simulink model "BodyMPC"  (R2023b)
settings: Solver=daessc  StartTime=0.0  StopTime=10  FixedStep=0.01  RelTol=1e-3
values from neighbouring files (symbols this model uses):
  Q = blkdiag(Q, q)    [SolveMPC.m]
undefined symbols (not defined in the file or in its folder): dw_des, LFstates, LRstates, p_cur, p_des, px, py, pz, RFstates, RRstates, v_cur, v_des, vx, vy, vz, w, w_des, X, Y, Z
libraries: sm_lib x57, nesl_utility x47
(part 1 of 3)
settings Model: Creator=a123  LastModifiedBy=a123

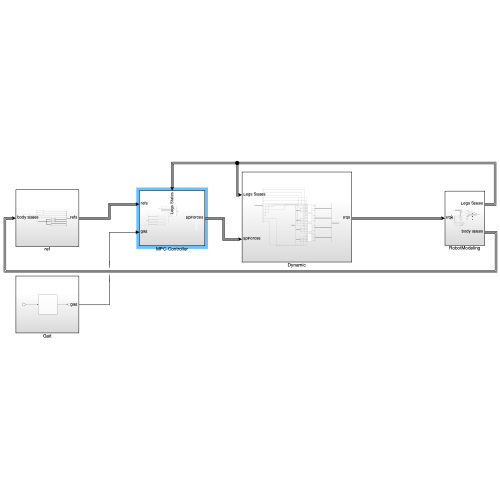
[thumbnail: Simulink's stored preview of the top-level diagram]
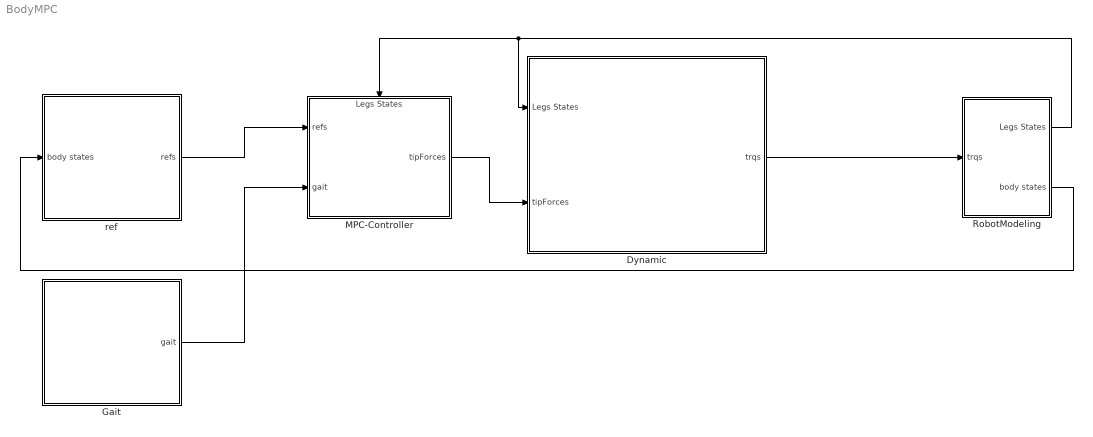
== system BodyMPC ==
  Dynamic : Subsystem
  Gait : Subsystem
  MPC-Controller : Subsystem
      settings: PortSchema="{\"entries\":[{\"content\":{\"sides\":[{\"content\":{\"connectorIds\":[\"In1\",\"In2\"]},\"type\":\"ConnectorPlacement.EquallySpacedRectSide\",\"uuid\":\"82207ac2-498d-428d-bb4d-b0457fff2070\"},{\"content\":{\"connectorIds\":[\"Out1\"],\"side\":\"RIGHT\"},\"type\":\"ConnectorPlacement.EquallySpacedRectSide\",\"uuid\":\"62017463-8491-4b37-95c8-f619666068a7\"},{\"content\":{\"connectorIds\":[\"In3\"],\"side\":\"TOP\"},\"type\":\"ConnectorPlacement.EquallySpacedRectSide\",\"uuid\":\"cf9993cf-df0f-41a3-a963-d91c0f700b7a\"}]},\"type\":\"ConnectorPlacement.EquallySpacedConnector\",\"uuid\":\"3cbcd1c8-4438-4464-bb77-c195fb75fbb3\"}],\"packageUris\":[\"http://schema.mathworks.com/mf0/Connector/R2020b\"],\"version\":\"1.0\"}"
  RobotModeling : Subsystem
  ref : Subsystem
  wires:
  RobotModeling/2(" body states") -> ref/1(body states)
  Dynamic/1(trqs) -> RobotModeling/1(trqs)
  RobotModeling/1(Legs States) -> MPC-Controller/3(Legs States), Dynamic/1(Legs States)
  ref/1(refs) -> MPC-Controller/1(refs)
  Gait/1(gait) -> MPC-Controller/2(gait)
  MPC-Controller/1(tipForces) -> Dynamic/2(tipForces)

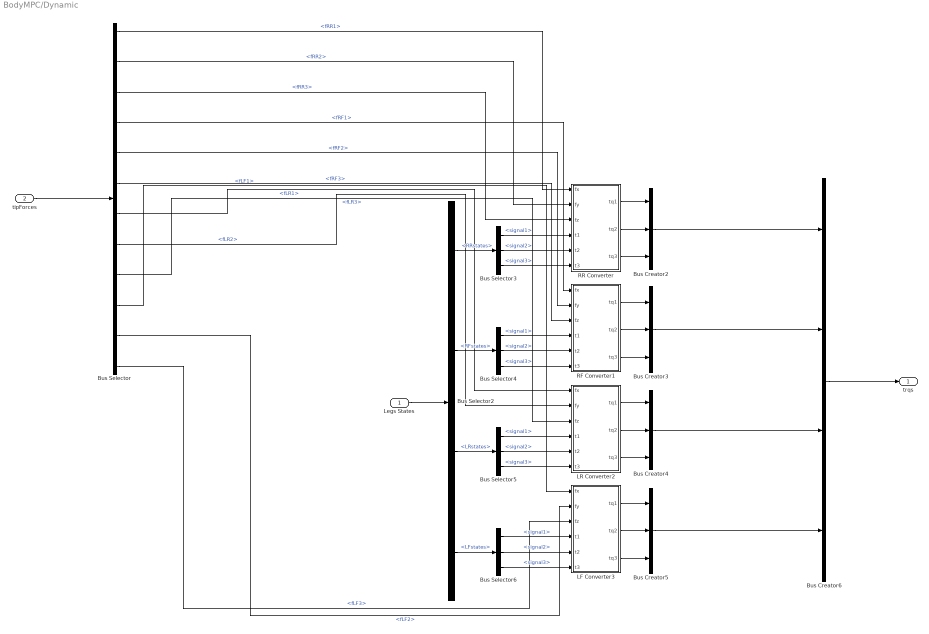
== system BodyMPC/Dynamic ==
  Legs States : Inport
  tipForces : Inport  Port=2
  Bus Creator{2..5} (4 alike) : BusCreator  Inputs=3
  Bus Creator6 : BusCreator  Inputs=4
  Bus Selector : BusSelector  OutputSignals=fRR1,fRR2,fRR3,fRF1,fRF2,fRF3,fLR1,fLR2,fLR3,fLF1,fLF2,fLF3
  Bus Selector2 : BusSelector  OutputSignals=RRstates,RFstates,LRstates,LFstates
  Bus Selector{3..6} (4 alike) : BusSelector  OutputSignals=signal1,signal2,signal3
  LF Converter3 : MATLAB Function  TreatAsAtomicUnit=on
  LR Converter2 : MATLAB Function  TreatAsAtomicUnit=on
  RF Converter1 : MATLAB Function  TreatAsAtomicUnit=on
  RR Converter : MATLAB Function  TreatAsAtomicUnit=on
  trqs : Outport
  wires:
  Bus Creator2/1 -> Bus Creator6/1
  Bus Creator3/1 -> Bus Creator6/2
  Bus Creator4/1 -> Bus Creator6/3
  Bus Creator5/1 -> Bus Creator6/4
  Bus Creator6/1 -> trqs/1
  Legs States/1 -> Bus Selector2/1
  Bus Selector2/1 -> Bus Selector3/1  "<RRstates>"
  Bus Selector3/1 -> RR Converter/4(t1)  "<signal1>"
  Bus Selector3/2 -> RR Converter/5(t2)  "<signal2>"
  Bus Selector3/3 -> RR Converter/6(t3)  "<signal3>"
  Bus Selector2/2 -> Bus Selector4/1  "<RFstates>"
  Bus Selector2/3 -> Bus Selector5/1  "<LRstates>"
  Bus Selector2/4 -> Bus Selector6/1  "<LFstates>"
  Bus Selector4/1 -> RF Converter1/4(t1)  "<signal1>"
  Bus Selector4/2 -> RF Converter1/5(t2)  "<signal2>"
  Bus Selector4/3 -> RF Converter1/6(t3)  "<signal3>"
  Bus Selector5/1 -> LR Converter2/4(t1)  "<signal1>"
  Bus Selector5/2 -> LR Converter2/5(t2)  "<signal2>"
  Bus Selector5/3 -> LR Converter2/6(t3)  "<signal3>"
  Bus Selector6/1 -> LF Converter3/4(t1)  "<signal1>"
  Bus Selector6/2 -> LF Converter3/5(t2)  "<signal2>"
  Bus Selector6/3 -> LF Converter3/6(t3)  "<signal3>"
  RR Converter/3(tq3) -> Bus Creator2/3
  RR Converter/2(tq2) -> Bus Creator2/2
  RR Converter/1(tq1) -> Bus Creator2/1
  RF Converter1/1(tq1) -> Bus Creator3/1
  RF Converter1/2(tq2) -> Bus Creator3/2
  RF Converter1/3(tq3) -> Bus Creator3/3
  LR Converter2/1(tq1) -> Bus Creator4/1
  LR Converter2/2(tq2) -> Bus Creator4/2
  LR Converter2/3(tq3) -> Bus Creator4/3
  LF Converter3/1(tq1) -> Bus Creator5/1
  LF Converter3/2(tq2) -> Bus Creator5/2
  LF Converter3/3(tq3) -> Bus Creator5/3
  tipForces/1 -> Bus Selector/1
  Bus Selector/1 -> RR Converter/1(fx)  "<fRR1>"
  Bus Selector/2 -> RR Converter/2(fy)  "<fRR2>"
  Bus Selector/3 -> RR Converter/3(fz)  "<fRR3>"
  Bus Selector/4 -> RF Converter1/1(fx)  "<fRF1>"
  Bus Selector/5 -> RF Converter1/2(fy)  "<fRF2>"
  Bus Selector/6 -> RF Converter1/3(fz)  "<fRF3>"
  Bus Selector/7 -> LR Converter2/1(fx)  "<fLR1>"
  Bus Selector/8 -> LR Converter2/2(fy)  "<fLR2>"
  Bus Selector/9 -> LR Converter2/3(fz)  "<fLR3>"
  Bus Selector/10 -> LF Converter3/1(fx)  "<fLF1>"
  Bus Selector/11 -> LF Converter3/2(fy)  "<fLF2>"
  Bus Selector/12 -> LF Converter3/3(fz)  "<fLF3>"

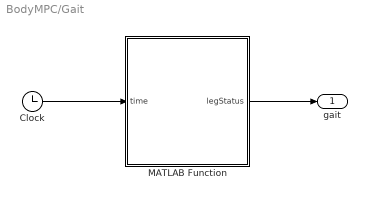
== system BodyMPC/Gait ==
  Clock : Clock
  MATLAB Function : MATLAB Function  TreatAsAtomicUnit=on
  gait : Outport
  wires:
  Clock/1 -> MATLAB Function/1(time)
  MATLAB Function/1(legStatus) -> gait/1

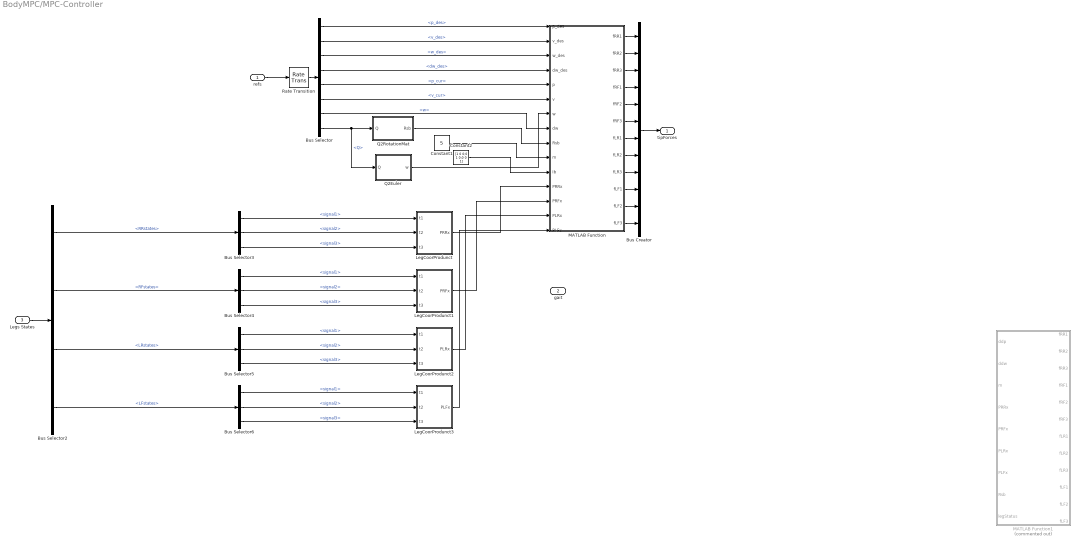
== system BodyMPC/MPC-Controller ==
  refs : Inport
  gait : Inport  Port=2
  Legs States : Inport  Port=3
  Bus Creator : BusCreator  Inputs=12
  Bus Selector : BusSelector  OutputSignals=p_des,v_des,w_des,dw_des,p_cur,v_cur,w,Q
  Bus Selector2 : BusSelector  OutputSignals=RRstates,RFstates,LRstates,LFstates
  Bus Selector{3..6} (4 alike) : BusSelector  OutputSignals=signal1,signal2,signal3
  Constant1 : Constant  Value=5
  Constant2 : Constant  Value=[1 0 0;0 1 0;0 0 1]
  LegCoorProdunct : MATLAB Function  TreatAsAtomicUnit=on
  LegCoorProdunct1 : MATLAB Function  TreatAsAtomicUnit=on
  LegCoorProdunct2 : MATLAB Function  TreatAsAtomicUnit=on
  LegCoorProdunct3 : MATLAB Function  TreatAsAtomicUnit=on
  MATLAB Function : MATLAB Function  TreatAsAtomicUnit=on
  MATLAB Function1 : MATLAB Function  Commented=on  TreatAsAtomicUnit=on
  Q2Euler : MATLAB Function  TreatAsAtomicUnit=on
  Q2RotationMat : MATLAB Function  TreatAsAtomicUnit=on
  Rate Transition : RateTransition  OutPortSampleTime=0.001
  tipForces : Outport
  wires:
  refs/1 -> Rate Transition/1
  Bus Selector/1 -> MATLAB Function/1(p_des)  "<p_des>"
  Bus Selector/2 -> MATLAB Function/2(v_des)  "<v_des>"
  Bus Selector/3 -> MATLAB Function/3(w_des)  "<w_des>"
  Bus Selector/4 -> MATLAB Function/4(dw_des)  "<dw_des>"
  Bus Selector/5 -> MATLAB Function/5(p)  "<p_cur>"
  Bus Selector/6 -> MATLAB Function/6(v)  "<v_cur>"
  Bus Selector/7 -> MATLAB Function/8(dw)  "<w>"
  Bus Selector/8 -> Q2Euler/1(Q), Q2RotationMat/1(Q)  "<Q>"
  Bus Selector5/2 -> LegCoorProdunct2/2(t2)  "<signal2>"
  Bus Selector5/3 -> LegCoorProdunct2/3(t3)  "<signal3>"
  Bus Selector6/3 -> LegCoorProdunct3/3(t3)  "<signal3>"
  Bus Selector2/3 -> Bus Selector5/1  "<LRstates>"
  Bus Selector6/1 -> LegCoorProdunct3/1(t1)  "<signal1>"
  Bus Selector4/2 -> LegCoorProdunct1/2(t2)  "<signal2>"
  Bus Selector6/2 -> LegCoorProdunct3/2(t2)  "<signal2>"
  Bus Selector3/2 -> LegCoorProdunct/2(t2)  "<signal2>"
  Bus Selector5/1 -> LegCoorProdunct2/1(t1)  "<signal1>"
  Bus Selector2/2 -> Bus Selector4/1  "<RFstates>"
  Bus Selector2/1 -> Bus Selector3/1  "<RRstates>"
  Legs States/1 -> Bus Selector2/1
  Bus Selector3/3 -> LegCoorProdunct/3(t3)  "<signal3>"
  Bus Selector4/1 -> LegCoorProdunct1/1(t1)  "<signal1>"
  Bus Selector3/1 -> LegCoorProdunct/1(t1)  "<signal1>"
  Bus Selector4/3 -> LegCoorProdunct1/3(t3)  "<signal3>"
  Bus Selector2/4 -> Bus Selector6/1  "<LFstates>"
  Bus Creator/1 -> tipForces/1
  Q2RotationMat/1(Rsb) -> MATLAB Function/9(Rsb)
  Constant1/1 -> MATLAB Function/10(m)
  Constant2/1 -> MATLAB Function/11(Ib)
  LegCoorProdunct/1(PRRx) -> MATLAB Function/12(PRRx)
  LegCoorProdunct1/1(PRFx) -> MATLAB Function/13(PRFx)
  LegCoorProdunct2/1(PLRx) -> MATLAB Function/14(PLRx)
  LegCoorProdunct3/1(PLFx) -> MATLAB Function/15(PLFx)
  MATLAB Function/1(fRR1) -> Bus Creator/1
  MATLAB Function/2(fRR2) -> Bus Creator/2
  MATLAB Function/3(fRR3) -> Bus Creator/3
  MATLAB Function/4(fRF1) -> Bus Creator/4
  MATLAB Function/5(fRF2) -> Bus Creator/5
  MATLAB Function/6(fRF3) -> Bus Creator/6
  MATLAB Function/7(fLR1) -> Bus Creator/7
  MATLAB Function/8(fLR2) -> Bus Creator/8
  MATLAB Function/9(fLR3) -> Bus Creator/9
  MATLAB Function/10(fLF1) -> Bus Creator/10
  MATLAB Function/11(fLF2) -> Bus Creator/11
  MATLAB Function/12(fLF3) -> Bus Creator/12
  Rate Transition/1 -> Bus Selector/1
  Q2Euler/1(w) -> MATLAB Function/7(w)

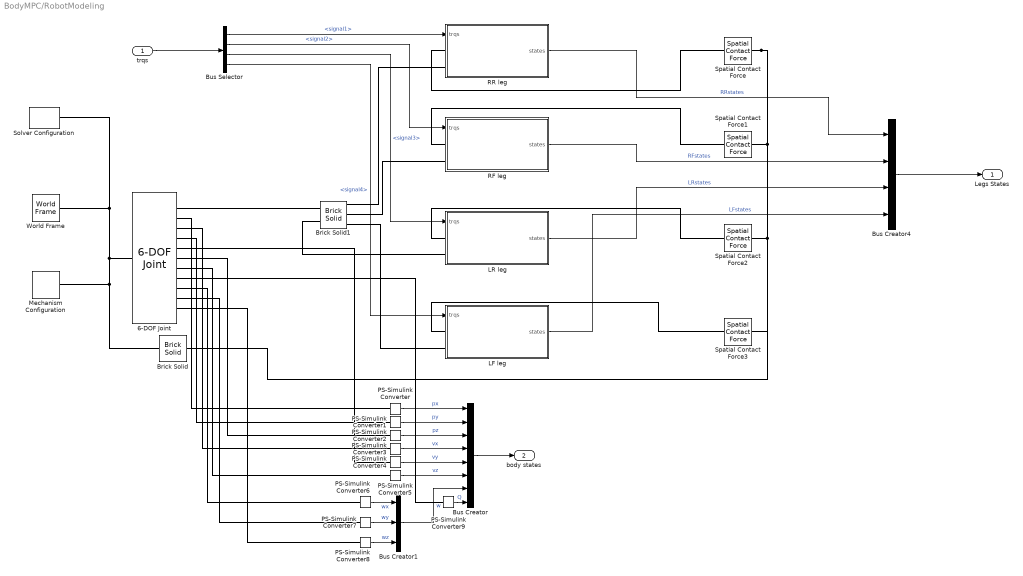
== system BodyMPC/RobotModeling ==
  trqs : Inport
  6-DOF Joint : sm_lib/Joints/6-DOF Joint  JointMode=Normal  SenseConstraintForce=off  SenseConstraintForceX=off  SenseConstraintForceY=off  SenseConstraintForceZ=off  SenseConstraintTorque=off  SenseConstraintTorqueX=off  SenseConstraintTorqueY=off  SenseConstraintTorqueZ=off  SenseTotalForce=off  SenseTotalForceX=off  SenseTotalForceY=off  SenseTotalForceZ=off  SenseTotalTorque=off  SenseTotalTorqueX=off  SenseTotalTorqueY=off  SenseTotalTorqueZ=off  CompositeWrenchDir=FollowerOnBase  CompositeWrenchFrame=BaseFrame  PxEquilibriumPosition=0  PxEquilibriumPositionUnits=m  PxSpringStiffness=0  PxSpringStiffnessUnits=N/m  PxDampingCoefficient=0  PxDampingCoefficientUnits=N/(m/s)  PxTorqueActuationMode=NoTorque  PxMotionActuationMode=ComputedMotion  PxSensePosition=on  PxSenseVelocity=on  PxSenseAcceleration=off  PxSenseTorqueForce=off  PxSenseLowerLimitTorqueForce=off  PxSenseUpperLimitTorqueForce=off  PxLowerLimitSpecify=off  PxLowerLimitBound=-1  PxLowerLimitBoundUnits=m  PxLowerLimitStiffness=1e6  PxLowerLimitStiffnessUnits=N/m  PxLowerLimitDamping=1e3  PxLowerLimitDampingUnits=N/(m/s)  PxLowerLimitTransitionRegionWidth=1e-4  PxLowerLimitTransitionRegionWidthUnits=m  PxUpperLimitSpecify=off  PxUpperLimitBound=1  PxUpperLimitBoundUnits=m  PxUpperLimitStiffness=1e6  PxUpperLimitStiffnessUnits=N/m  PxUpperLimitDamping=1e3  PxUpperLimitDampingUnits=N/(m/s)  PxUpperLimitTransitionRegionWidth=1e-4  PxUpperLimitTransitionRegionWidthUnits=m  PxPositionTargetSpecify=off  PxPositionTargetPriority=High  PxPositionTargetValue=0  PxPositionTargetValueUnits=m  PxVelocityTargetSpecify=off  PxVelocityTargetPriority=High  PxVelocityTargetValue=0  PxVelocityTargetValueUnits=m/s  PyEquilibriumPosition=0  PyEquilibriumPositionUnits=m  PySpringStiffness=0  PySpringStiffnessUnits=N/m  PyDampingCoefficient=0  PyDampingCoefficientUnits=N/(m/s)  PyTorqueActuationMode=NoTorque  PyMotionActuationMode=ComputedMotion  PySensePosition=on  PySenseVelocity=on  PySenseAcceleration=off  PySenseTorqueForce=off  PySenseLowerLimitTorqueForce=off  PySenseUpperLimitTorqueForce=off  PyLowerLimitSpecify=off  PyLowerLimitBound=-1  PyLowerLimitBoundUnits=m  PyLowerLimitStiffness=1e6  PyLowerLimitStiffnessUnits=N/m  PyLowerLimitDamping=1e3  PyLowerLimitDampingUnits=N/(m/s)  PyLowerLimitTransitionRegionWidth=1e-4  PyLowerLimitTransitionRegionWidthUnits=m  PyUpperLimitSpecify=off  PyUpperLimitBound=1  PyUpperLimitBoundUnits=m  PyUpperLimitStiffness=1e6  PyUpperLimitStiffnessUnits=N/m  PyUpperLimitDamping=1e3  PyUpperLimitDampingUnits=N/(m/s)  PyUpperLimitTransitionRegionWidth=1e-4  PyUpperLimitTransitionRegionWidthUnits=m  PyPositionTargetSpecify=on  PyPositionTargetPriority=High  PyPositionTargetValue=1.7  PyPositionTargetValueUnits=m  PyVelocityTargetSpecify=off  PyVelocityTargetPriority=High  PyVelocityTargetValue=0  PyVelocityTargetValueUnits=m/s  PzEquilibriumPosition=0  PzEquilibriumPositionUnits=m  PzSpringStiffness=0  PzSpringStiffnessUnits=N/m  PzDampingCoefficient=0  PzDampingCoefficientUnits=N/(m/s)  PzTorqueActuationMode=NoTorque  PzMotionActuationMode=ComputedMotion  PzSensePosition=on  PzSenseVelocity=on  PzSenseAcceleration=off  PzSenseTorqueForce=off  PzSenseLowerLimitTorqueForce=off  PzSenseUpperLimitTorqueForce=off  PzLowerLimitSpecify=off  PzLowerLimitBound=-1  PzLowerLimitBoundUnits=m  PzLowerLimitStiffness=1e6  PzLowerLimitStiffnessUnits=N/m  PzLowerLimitDamping=1e3  PzLowerLimitDampingUnits=N/(m/s)  PzLowerLimitTransitionRegionWidth=1e-4  PzLowerLimitTransitionRegionWidthUnits=m  PzUpperLimitSpecify=off  PzUpperLimitBound=1  PzUpperLimitBoundUnits=m  PzUpperLimitStiffness=1e6  PzUpperLimitStiffnessUnits=N/m  PzUpperLimitDamping=1e3  PzUpperLimitDampingUnits=N/(m/s)  PzUpperLimitTransitionRegionWidth=1e-4  PzUpperLimitTransitionRegionWidthUnits=m  PzPositionTargetSpecify=off  PzPositionTargetPriority=High  PzPositionTargetValue=0  PzPositionTargetValueUnits=m  PzVelocityTargetSpecify=off  PzVelocityTargetPriority=High  PzVelocityTargetValue=0  PzVelocityTargetValueUnits=m/s  SphEqPosRotationMethod=None  SphEqPosRotationAngleUnits=deg  SphEqPosRotationStandardAxis=+Z  SphEqPosRotationAngle=0.0  SphEqPosRotationArbitraryAxis=[0 0 1]  SphEqPosFollAlignAxisA=+X  SphEqPosBaseAlignAxisA=+Y  SphEqPosFollAlignAxisB=+Y  SphEqPosBaseAlignAxisB=+Z  SphEqPosRotationSequenceAxes=FollowerAxes  SphEqPosRotationSequence=XYX  SphEqPosRotationSequenceAngles=[0 0 0]  SphEqPosRotationSequenceAnglesUnits=deg  SphEqPosRotationMatrix=[1 0 0; 0 1 0; 0 0 1]  SphEqPosQuaternion=[1 0 0 0]  SphSpringStiffness=0  SphSpringStiffnessUnits=N*m/deg  SphDampingCoefficient=0  SphDampingCoefficientUnits=N*m/(deg/s)  SphActuateTorqueX=off  SphActuateTorqueY=off  SphActuateTorqueZ=off  SphActuateTorque=off  SphTorqueActuationMode=NoTorque  SphMotionActuationMode=ComputedMotion  SphActuationFrame=BaseFrame  SphSensePosition=on  SphSenseVelocityX=on  SphSenseVelocityY=on  SphSenseVelocityZ=on  SphSenseVelocity=off  SphSenseAccelerationX=off  SphSenseAccelerationY=off  SphSenseAccelerationZ=off  SphSenseAcceleration=off  SphSenseTorqueX=off  SphSenseTorqueY=off  SphSenseTorqueZ=off  SphSenseTorqueForce=off  SphSenseLowerLimitTorqueMag=off  SphSenseUpperLimitTorqueMag=off  SphSensingFrame=BaseFrame  SphLowerLimitSpecify=off  SphLowerLimitBound=15  SphLowerLimitBoundUnits=deg  SphLowerLimitStiffness=1e4  SphLowerLimitStiffnessUnits=N*m/deg  SphLowerLimitDamping=10  SphLowerLimitDampingUnits=N*m/(deg/s)  SphLowerLimitTransitionRegionWidth=0.1  SphLowerLimitTransitionRegionWidthUnits=deg  SphUpperLimitSpecify=off  SphUpperLimitBound=45  SphUpperLimitBoundUnits=deg  SphUpperLimitStiffness=1e4  SphUpperLimitStiffnessUnits=N*m/deg  SphUpperLimitDamping=10  SphUpperLimitDampingUnits=N*m/(deg/s)  SphUpperLimitTransitionRegionWidth=0.1  SphUpperLimitTransitionRegionWidthUnits=deg  SphPositionTargetRotationMethod=Quaternion  SphPositionTargetRotationAngleUnits=deg  SphPositionTargetRotationStandardAxis=+Z  SphPositionTargetRotationAngle=0.0  SphPositionTargetRotationArbitraryAxis=[0 0 1]  SphPositionTargetFollAlignAxisA=+X  SphPositionTargetBaseAlignAxisA=+Y  SphPositionTargetFollAlignAxisB=+Y  SphPositionTargetBaseAlignAxisB=+Z  SphPositionTargetRotationSequenceAxes=FollowerAxes  SphPositionTargetRotationSequence=XYX  SphPositionTargetRotationSequenceAngles=[0 0 0]  SphPositionTargetRotationSequenceAnglesUnits=deg  SphPositionTargetRotationMatrix=[1 0 0; 0 1 0; 0 0 1]  SphPositionTargetQuaternion=[0.9 0 0 0]  SphPositionTargetSpecify=off  SphPositionTargetPriority=High  SphVelocityTargetValue=[0 0 0]  SphVelocityTargetValueUnits=deg/s  SphVelocityTargetSpecify=off  SphVelocityTargetPriority=High  SphVelocityTargetInFollowerFrame=on
  Brick Solid : sm_lib/Body Elements/Brick Solid  GraphicAmbientColor=[0.15 0.15 0.15 1.0]  BasedOnType=Density  BrickDimensions=[20 0.01 20]  BrickDimensionsUnits=m  CenterOfMass=[0 0 0]  CenterOfMassUnits=m  GraphicDiffuseColor=[0.5 0.5 0.5]  Density=1000  DensityUnits=kg/m^3  DoExposeReferenceFrame=on  GraphicEmissiveColor=[0.0 0.0 0.0 1.0]  ExportEntireGeometry=on  SerializedFrames=<Frames/>  MarkerShape=Sphere  MarkerSize=10  GraphicType=FromGeometry  InertiaType=CalculateFromGeometry  Mass=1  MassUnits=kg  MomentsOfInertia=[1 1 1]  MomentsOfInertiaUnits=kg*m^2  GraphicOpacity=1.0  ProductsOfInertia=[0 0 0]  ProductsOfInertiaUnits=kg*m^2  GraphicShininess=75  GraphicSpecularColor=[0.5 0.5 0.5 1.0]  GraphicVisPropType=SimpleVisualProperties
  Brick Solid1 : sm_lib/Body Elements/Brick Solid  GraphicAmbientColor=[0.15 0.15 0.15 1.0]  BasedOnType=Mass  BrickDimensions=[2.5 0.3 0.8]  BrickDimensionsUnits=m  CenterOfMass=[0 0 0]  CenterOfMassUnits=m  GraphicDiffuseColor=[1.0 0.6 0.2]  Density=1000  DensityUnits=kg/m^3  DoExposeReferenceFrame=on  GraphicEmissiveColor=[0.0 0.0 0.0 1.0]  ExportEntireGeometry=off  SerializedFrames=<Frames><Frame><Id>Frame1</Id><Value><Name>RR</Name><Origin><Source>ReferenceFrame</Source><FeatureName></FeatureName></Origin><PrimaryAxis><DefinedDirection>+Z</DefinedDirection><Source>ReferenceFrame</Source><SourceDirection>-X</SourceDirection><FeatureName></FeatureName></PrimaryAxis><SecondaryAxis><DefinedDirection>+X</DefinedDirection><Source>ReferenceFrame</Source><SourceDirection>+Z</SourceDirection><FeatureName></FeatureName></SecondaryAxis></Value></Frame><Frame><Id>Frame2</Id><Value><Name>RF</Name><Origin><Source>ReferenceFrame</Source><FeatureName></FeatureName></Origin><PrimaryAxis><DefinedDirection>+Z</DefinedDirection><Source>ReferenceFrame</Source><SourceDirection>-X</SourceDirection><FeatureName></FeatureName></PrimaryAxis><SecondaryAxis><DefinedDirection>+X</DefinedDirection><Source>ReferenceFrame</Source><SourceDirection>+Z</SourceDirection><FeatureName></FeatureName></SecondaryAxis></Value></Frame><Frame><Id>Frame3</Id><Value><Name>LR</Name><Origin><Source>ReferenceFrame</Source><FeatureName></FeatureName></Origin><PrimaryAxis><DefinedDirection>+Z</DefinedDirection><Source>ReferenceFrame</Source><SourceDirection>-X</SourceDirection><FeatureName></FeatureName></PrimaryAxis><SecondaryAxis><DefinedDirection>+X</DefinedDirection><Source>ReferenceFrame</Source><SourceDirection>+Z</SourceDirection><FeatureName></FeatureName></SecondaryAxis></Value></Frame><Frame><Id>Frame4</Id><Value><Name>LF</Name><Origin><Source>ReferenceFrame</Source><FeatureName></FeatureName></Origin><PrimaryAxis><DefinedDirection>+Z</DefinedDirection><Source>ReferenceFrame</Source><SourceDirection>-X</SourceDirection><FeatureName></FeatureName></PrimaryAxis><SecondaryAxis><DefinedDirection>+X</DefinedDirection><Source>ReferenceFrame</Source><SourceDirection>+Z</SourceDirection><FeatureName></FeatureName></SecondaryAxis></Value></Frame></Frames>  MarkerShape=Sphere  MarkerSize=10  GraphicType=FromGeometry  InertiaType=Custom  Mass=5  MassUnits=kg  MomentsOfInertia=[1 1 1]  MomentsOfInertiaUnits=kg*m^2  GraphicOpacity=1.0  ProductsOfInertia=[0 0 0]  ProductsOfInertiaUnits=kg*m^2  GraphicShininess=75  GraphicSpecularColor=[0.5 0.5 0.5 1.0]  GraphicVisPropType=SimpleVisualProperties
  Bus Creator : BusCreator  Inputs=px,py,pz,vx,vy,vz,w,Q
  Bus Creator1 : BusCreator  Inputs=3
  Bus Creator4 : BusCreator  Inputs=RRstates,RFstates,LRstates,LFstates
  Bus Selector : BusSelector  OutputSignals=signal1,signal2,signal3,signal4
  LF leg : Subsystem
  LR leg : Subsystem
  Mechanism Configuration : sm_lib/Utilities/Mechanism Configuration  UniformGravity=Constant  GravityVector=[0 -9.80665 0]  GravityVectorUnits=m/s^2  LinearizationDelta=0.001  JointModeTransitionNonlinearIterations=2
  PS-Simulink Converter{,1..9} (10 alike) : nesl_utility/PS-Simulink Converter  PhysicalDomain=network_engine_domain  SubClassName=ps_output  LeftPortType=input  RightPortType=output  PseudoPeriodic=off  Frequencies=[]  VectorFormat=inherit  Unit=inherit  AffineConversion=off
  RF leg : Subsystem
  RR leg : Subsystem
  Solver Configuration : nesl_utility/Solver Configuration  PhysicalDomain=network_engine_domain  SubClassName=solver  LeftPortType=input  RightPortType=generic  Tones=[]  Harmonics=[]  SimulateNoise=off  Profile=off  UseLocalSampling=off  EnableSwitchedLinearOptims=on  FrequencyDomain=off  UseCCode=off  RelTol=0.001  AbsTol=0.001  MinStep=1e-09  ToWorkspace=off  RevertToSquareIcSolve=off  NumHomotopyIterations=100  PhasorMode=off  PhasorModeNumHarmonics=1  ConsistencySolver=NEWTON_XTOL_AFTER_FTOL  IndexReductionMethod=DerivativeReplacement  DoDC=off  ResidualTolerance=1e-09  ConsistencyTolSource=GLOBAL  ConsistencyAbsTol=0.001  ConsistencyRelTol=0.001  ConsistencyTolFactor=0.001  UseLocalSolver=off  LocalSolverChoice=NE_BACKWARD_EULER_ADVANCER  ResolveIndetEquations=on  FunctionEvalNumThread=1  LocalSolverSampleTime=0.001  DoFixedCost=off  MaxNonlinIter=3  MaxModeIter=2  ComputeImpulses=off  ImpulseIterations=2  LinearAlgebra=auto  LinearAlgebraNumThread=0  EquationFormulation=NE_TIME_EF  DelaysMemoryBudget=1024  AutomaticFiltering=on  FilteringTimeConstant=0.001  PartitionStorageMethod=AS_NEEDED  PartitionMemoryBudget=1024  PartitionMethod=ROBUST  MultibodyUseLocalSolver=off  MultibodyLocalSolverChoice=ODE1  MultibodyLocalSolverSampleTime=0.001
  Spatial Contact Force{,1..3} (4 alike) : sm_lib/Forces and Torques/Spatial Contact Force  SenseContactBaseRotation=off  SenseContactBaseTranslation=off  CoefficientOfDynamicFriction=2  CoefficientOfStaticFriction=2  NormalDamping=1e3  NormalDampingUnits=N/(m/s)  SenseContactSignal=off  NormalStiffness=1e6  NormalStiffnessUnits=N/m  FrictionalCriticalVelocity=1e-3  FrictionalCriticalVelocityUnits=m/s  ZeroCrossDetectContactStartAndEnd=off  SenseContactFollowerRotation=off  SenseContactFollowerTranslation=off  FrictionType=SmoothStickSlip  SenseFrictionalForceMagnitude=off  SenseNormalForceMagnitude=off  NormalForceType=SmoothSpringDamper  SenseNormalVelocity=off  SensePenetrationDepth=off  SenseSeparationDistance=off  SenseTangentialVelocity=off  NormalTransitionRegionWidth=1e-4  NormalTransitionRegionWidthUnits=m
  World Frame : sm_lib/Frames and Transforms/World Frame
  Legs States : Outport
  " body states" : Outport  Port=2
  wires:
  Bus Creator4/1 -> Legs States/1
  trqs/1 -> Bus Selector/1
  Bus Selector/1 -> RR leg/1(trqs)  "<signal1>"
  Bus Selector/2 -> RF leg/1(trqs)  "<signal2>"
  Bus Selector/3 -> LR leg/1(trqs)  "<signal3>"
  Bus Selector/4 -> LF leg/1(trqs)  "<signal4>"
  RR leg/1(states) -> Bus Creator4/1  "RRstates"
  RF leg/1(states) -> Bus Creator4/2  "RFstates"
  LR leg/1(states) -> Bus Creator4/3  "LRstates"
  LF leg/1(states) -> Bus Creator4/4  "LFstates"
  PS-Simulink Converter/1 -> Bus Creator/1  "px"
  PS-Simulink Converter1/1 -> Bus Creator/2  "py"
  PS-Simulink Converter2/1 -> Bus Creator/3  "pz"
  PS-Simulink Converter3/1 -> Bus Creator/4  "vx"
  PS-Simulink Converter4/1 -> Bus Creator/5  "vy"
  PS-Simulink Converter5/1 -> Bus Creator/6  "vz"
  Bus Creator/1 -> " body states"/1
  PS-Simulink Converter8/1 -> Bus Creator1/3  "wz"
  PS-Simulink Converter7/1 -> Bus Creator1/2  "wy"
  PS-Simulink Converter6/1 -> Bus Creator1/1  "wx"
  Bus Creator1/1 -> Bus Creator/7  "w"
  PS-Simulink Converter9/1 -> Bus Creator/8  "Q"
  connections:
  Solver Configuration/RConn1 -- Mechanism Configuration/RConn1 -- Brick Solid/RConn1 -- 6-DOF Joint/LConn1 -- World Frame/RConn1
  Brick Solid1/RConn1 -- 6-DOF Joint/RConn1
  Spatial Contact Force/LConn1 -- RR leg/LConn1
  Spatial Contact Force/RConn1 -- Brick Solid/LConn1 -- Spatial Contact Force3/RConn1 -- Spatial Contact Force2/RConn1 -- Spatial Contact Force1/RConn1
  Brick Solid1/LConn1 -- RR leg/LConn2
  Brick Solid1/LConn2 -- RF leg/LConn2
  Brick Solid1/LConn3 -- LF leg/LConn2
  Brick Solid1/RConn2 -- LR leg/LConn2
  Spatial Contact Force1/LConn1 -- RF leg/LConn1
  Spatial Contact Force2/LConn1 -- LR leg/LConn1
  Spatial Contact Force3/LConn1 -- LF leg/LConn1
  6-DOF Joint/RConn2 -- PS-Simulink Converter/LConn1
  6-DOF Joint/RConn4 -- PS-Simulink Converter1/LConn1
  6-DOF Joint/RConn6 -- PS-Simulink Converter2/LConn1
  6-DOF Joint/RConn3 -- PS-Simulink Converter3/LConn1
  6-DOF Joint/RConn5 -- PS-Simulink Converter4/LConn1
  6-DOF Joint/RConn7 -- PS-Simulink Converter5/LConn1
  6-DOF Joint/RConn9 -- PS-Simulink Converter6/LConn1
  6-DOF Joint/RConn10 -- PS-Simulink Converter7/LConn1
  6-DOF Joint/RConn11 -- PS-Simulink Converter8/LConn1
  6-DOF Joint/RConn8 -- PS-Simulink Converter9/LConn1

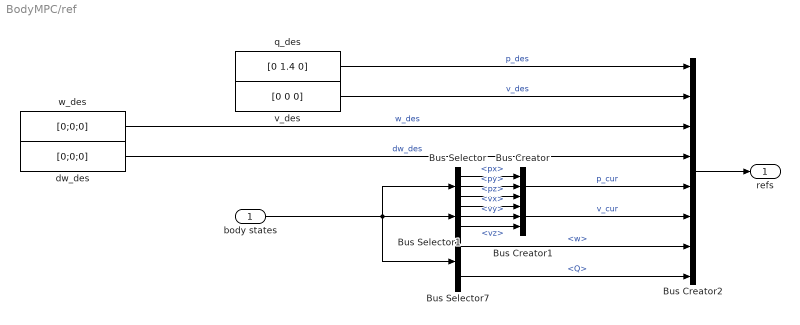
== system BodyMPC/ref ==
  body states : Inport
  Bus Creator : BusCreator  Inputs=3
  Bus Creator1 : BusCreator  Inputs=3
  Bus Creator2 : BusCreator  Inputs=p_des,v_des,w_des,dw_des,p_cur,v_cur,w,Q
  Bus Selector : BusSelector  OutputSignals=px,py,pz
  Bus Selector1 : BusSelector  OutputSignals=vx,vy,vz
  Bus Selector7 : BusSelector  OutputSignals=w,Q
  dw_des : Constant  Value=[0;0;0]  VectorParams1D=off
  q_des : Constant  Value=[0 1.4 0]
  v_des : Constant  Value=[0 0 0]
  w_des : Constant  Value=[0;0;0]  VectorParams1D=off
  refs : Outport
  wires:
  Bus Selector1/3 -> Bus Creator1/3  "<vz>"
  dw_des/1 -> Bus Creator2/4  "dw_des"
  Bus Selector1/2 -> Bus Creator1/2  "<vy>"
  q_des/1 -> Bus Creator2/1  "p_des"
  Bus Selector7/2 -> Bus Creator2/8  "<Q>"
  Bus Selector/3 -> Bus Creator/3  "<pz>"
  body states/1 -> Bus Selector7/1, Bus Selector1/1, Bus Selector/1
  Bus Selector1/1 -> Bus Creator1/1  "<vx>"
  v_des/1 -> Bus Creator2/2  "v_des"
  Bus Selector/1 -> Bus Creator/1  "<px>"
  Bus Creator/1 -> Bus Creator2/5  "p_cur"
  w_des/1 -> Bus Creator2/3  "w_des"
  Bus Selector/2 -> Bus Creator/2  "<py>"
  Bus Selector7/1 -> Bus Creator2/7  "<w>"
  Bus Creator1/1 -> Bus Creator2/6  "v_cur"
  Bus Creator2/1 -> refs/1

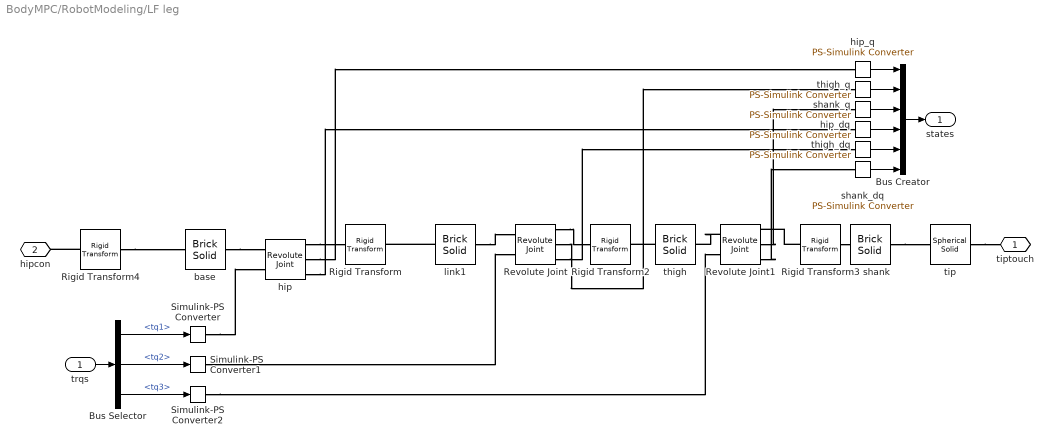
== system BodyMPC/RobotModeling/LF leg ==
  trqs : Inport
  Bus Creator : BusCreator  Inputs=6
  Bus Selector : BusSelector  OutputSignals=tq1,tq2,tq3
  Revolute Joint : sm_lib/Joints/Revolute Joint  JointMode=Normal  SenseConstraintForce=off  SenseConstraintForceX=off  SenseConstraintForceY=off  SenseConstraintForceZ=off  SenseConstraintTorque=off  SenseConstraintTorqueX=off  SenseConstraintTorqueY=off  SenseConstraintTorqueZ=off  SenseTotalForce=off  SenseTotalForceX=off  SenseTotalForceY=off  SenseTotalForceZ=off  SenseTotalTorque=off  SenseTotalTorqueX=off  SenseTotalTorqueY=off  SenseTotalTorqueZ=off  CompositeWrenchDir=FollowerOnBase  CompositeWrenchFrame=BaseFrame  EquilibriumPosition=0  EquilibriumPositionUnits=deg  SpringStiffness=0  SpringStiffnessUnits=N*m/deg  DampingCoefficient=0  DampingCoefficientUnits=N*m/(deg/s)  TorqueActuationMode=InputTorque  MotionActuationMode=ComputedMotion  SensePosition=on  SenseVelocity=on  SenseAcceleration=off  SenseTorqueForce=off  SenseLowerLimitTorqueForce=off  SenseUpperLimitTorqueForce=off  LowerLimitSpecify=off  LowerLimitBound=-90  LowerLimitBoundUnits=deg  LowerLimitStiffness=1e4  LowerLimitStiffnessUnits=N*m/deg  LowerLimitDamping=10  LowerLimitDampingUnits=N*m/(deg/s)  LowerLimitTransitionRegionWidth=0.1  LowerLimitTransitionRegionWidthUnits=deg  UpperLimitSpecify=off  UpperLimitBound=90  UpperLimitBoundUnits=deg  UpperLimitStiffness=1e4  UpperLimitStiffnessUnits=N*m/deg  UpperLimitDamping=10  UpperLimitDampingUnits=N*m/(deg/s)  UpperLimitTransitionRegionWidth=0.1  UpperLimitTransitionRegionWidthUnits=deg  PositionTargetSpecify=off  PositionTargetPriority=High  PositionTargetValue=0  PositionTargetValueUnits=deg  VelocityTargetSpecify=off  VelocityTargetPriority=High  VelocityTargetValue=0  VelocityTargetValueUnits=deg/s
  Revolute Joint1 : sm_lib/Joints/Revolute Joint  JointMode=Normal  SenseConstraintForce=off  SenseConstraintForceX=off  SenseConstraintForceY=off  SenseConstraintForceZ=off  SenseConstraintTorque=off  SenseConstraintTorqueX=off  SenseConstraintTorqueY=off  SenseConstraintTorqueZ=off  SenseTotalForce=off  SenseTotalForceX=off  SenseTotalForceY=off  SenseTotalForceZ=off  SenseTotalTorque=off  SenseTotalTorqueX=off  SenseTotalTorqueY=off  SenseTotalTorqueZ=off  CompositeWrenchDir=FollowerOnBase  CompositeWrenchFrame=BaseFrame  EquilibriumPosition=0  EquilibriumPositionUnits=deg  SpringStiffness=0  SpringStiffnessUnits=N*m/deg  DampingCoefficient=0  DampingCoefficientUnits=N*m/(deg/s)  TorqueActuationMode=InputTorque  MotionActuationMode=ComputedMotion  SensePosition=on  SenseVelocity=on  SenseAcceleration=off  SenseTorqueForce=off  SenseLowerLimitTorqueForce=off  SenseUpperLimitTorqueForce=off  LowerLimitSpecify=off  LowerLimitBound=-90  LowerLimitBoundUnits=deg  LowerLimitStiffness=1e4  LowerLimitStiffnessUnits=N*m/deg  LowerLimitDamping=10  LowerLimitDampingUnits=N*m/(deg/s)  LowerLimitTransitionRegionWidth=0.1  LowerLimitTransitionRegionWidthUnits=deg  UpperLimitSpecify=off  UpperLimitBound=90  UpperLimitBoundUnits=deg  UpperLimitStiffness=1e4  UpperLimitStiffnessUnits=N*m/deg  UpperLimitDamping=10  UpperLimitDampingUnits=N*m/(deg/s)  UpperLimitTransitionRegionWidth=0.1  UpperLimitTransitionRegionWidthUnits=deg  PositionTargetSpecify=off  PositionTargetPriority=High  PositionTargetValue=20  PositionTargetValueUnits=deg  VelocityTargetSpecify=off  VelocityTargetPriority=High  VelocityTargetValue=0  VelocityTargetValueUnits=deg/s
  Rigid Transform : sm_lib/Frames and Transforms/Rigid Transform  TranslationMethod=Cartesian  TranslationStandardOffset=0  TranslationStandardOffsetUnits=m  TranslationStandardAxis=+Z  TranslationCartesianOffset=[0.1 0 0]  TranslationCartesianOffsetUnits=m  TranslationROffset=0  TranslationROffsetUnits=m  TranslationZOffset=0  TranslationZOffsetUnits=m  TranslationThetaOffset=0  TranslationThetaOffsetUnits=deg  RotationMethod=None  RotationAngleUnits=deg  RotationStandardAxis=+Z  RotationAngle=0.0  RotationArbitraryAxis=[0 0 1]  FollAlignAxisA=+X  BaseAlignAxisA=+Y  FollAlignAxisB=+Y  BaseAlignAxisB=+Z  RotationSequenceAxes=FollowerAxes  RotationSequence=XYX  RotationSequenceAngles=[0 0 0]  RotationSequenceAnglesUnits=deg  RotationMatrix=[1 0 0; 0 1 0; 0 0 1]  Quaternion=[1 0 0 0]
  Rigid Transform2 : sm_lib/Frames and Transforms/Rigid Transform  TranslationMethod=Cartesian  TranslationStandardOffset=0  TranslationStandardOffsetUnits=m  TranslationStandardAxis=+Z  TranslationCartesianOffset=[0 -0.4 0]  TranslationCartesianOffsetUnits=m  TranslationROffset=0  TranslationROffsetUnits=m  TranslationZOffset=0  TranslationZOffsetUnits=m  TranslationThetaOffset=0  TranslationThetaOffsetUnits=deg  RotationMethod=None  RotationAngleUnits=deg  RotationStandardAxis=+Z  RotationAngle=0.0  RotationArbitraryAxis=[0 0 1]  FollAlignAxisA=+X  BaseAlignAxisA=+Y  FollAlignAxisB=+Y  BaseAlignAxisB=+Z  RotationSequenceAxes=FollowerAxes  RotationSequence=XYX  RotationSequenceAngles=[0 0 0]  RotationSequenceAnglesUnits=deg  RotationMatrix=[1 0 0; 0 1 0; 0 0 1]  Quaternion=[1 0 0 0]
  Rigid Transform3 : sm_lib/Frames and Transforms/Rigid Transform  TranslationMethod=Cartesian  TranslationStandardOffset=0  TranslationStandardOffsetUnits=m  TranslationStandardAxis=+Z  TranslationCartesianOffset=[0 -0.4 0]  TranslationCartesianOffsetUnits=m  TranslationROffset=0  TranslationROffsetUnits=m  TranslationZOffset=0  TranslationZOffsetUnits=m  TranslationThetaOffset=0  TranslationThetaOffsetUnits=deg  RotationMethod=None  RotationAngleUnits=deg  RotationStandardAxis=+Z  RotationAngle=0.0  RotationArbitraryAxis=[0 0 1]  FollAlignAxisA=+X  BaseAlignAxisA=+Y  FollAlignAxisB=+Y  BaseAlignAxisB=+Z  RotationSequenceAxes=FollowerAxes  RotationSequence=XYX  RotationSequenceAngles=[0 0 0]  RotationSequenceAnglesUnits=deg  RotationMatrix=[1 0 0; 0 1 0; 0 0 1]  Quaternion=[1 0 0 0]
  Rigid Transform4 : sm_lib/Frames and Transforms/Rigid Transform  TranslationMethod=Cartesian  TranslationStandardOffset=0  TranslationStandardOffsetUnits=m  TranslationStandardAxis=+Z  TranslationCartesianOffset=[-0.35 0 -1.25]  TranslationCartesianOffsetUnits=m  TranslationROffset=0  TranslationROffsetUnits=m  TranslationZOffset=0  TranslationZOffsetUnits=m  TranslationThetaOffset=0  TranslationThetaOffsetUnits=deg  RotationMethod=StandardAxis  RotationAngleUnits=deg  RotationStandardAxis=+Y  RotationAngle=270  RotationArbitraryAxis=[0 0 1]  FollAlignAxisA=+X  BaseAlignAxisA=+Y  FollAlignAxisB=+Y  BaseAlignAxisB=+Z  RotationSequenceAxes=FollowerAxes  RotationSequence=XYX  RotationSequenceAngles=[0 0 0]  RotationSequenceAnglesUnits=deg  RotationMatrix=[1 0 0; 0 1 0; 0 0 1]  Quaternion=[1 0 0 0]
  Simulink-PS Converter : nesl_utility/Simulink-PS Converter  PhysicalDomain=network_engine_domain  SubClassName=ps_input  LeftPortType=input  RightPortType=output  PseudoPeriodic=off  Frequencies=[]  NoiseDistribution=none  NoiseParameters=[]  Unit=1  AffineConversion=off  FilteringAndDerivatives=provide  SimscapeFilterOrder=1  InputFilterTimeConstant=0.001  UdotUserProvided=0
  Simulink-PS Converter1 : nesl_utility/Simulink-PS Converter  PhysicalDomain=network_engine_domain  SubClassName=ps_input  LeftPortType=input  RightPortType=output  PseudoPeriodic=off  Frequencies=[]  NoiseDistribution=none  NoiseParameters=[]  Unit=1  AffineConversion=off  FilteringAndDerivatives=provide  SimscapeFilterOrder=1  InputFilterTimeConstant=0.001  UdotUserProvided=0
  Simulink-PS Converter2 : nesl_utility/Simulink-PS Converter  PhysicalDomain=network_engine_domain  SubClassName=ps_input  LeftPortType=input  RightPortType=output  PseudoPeriodic=off  Frequencies=[]  NoiseDistribution=none  NoiseParameters=[]  Unit=1  AffineConversion=off  FilteringAndDerivatives=provide  SimscapeFilterOrder=1  InputFilterTimeConstant=0.001  UdotUserProvided=0
  base : sm_lib/Body Elements/Brick Solid  GraphicAmbientColor=[0.15 0.15 0.15 1.0]  BasedOnType=Density  BrickDimensions=[0.05 0.05 0.05]  BrickDimensionsUnits=m  CenterOfMass=[0 0 0]  CenterOfMassUnits=m  GraphicDiffuseColor=[0.0 0.8 0.8]  Density=1000  DensityUnits=kg/m^3  DoExposeReferenceFrame=on  GraphicEmissiveColor=[0.0 0.0 0.0 1.0]  ExportEntireGeometry=off  SerializedFrames=<Frames><Frame><Id>Frame1</Id><Value><Name>hip</Name><Origin><Source>GeometricFeature</Source><FeatureName>+z surface</FeatureName></Origin><PrimaryAxis><DefinedDirection>+Z</DefinedDirection><Source>ReferenceFrame</Source><SourceDirection>-X</SourceDirection><FeatureName></FeatureName></PrimaryAxis><SecondaryAxis><DefinedDirection>+X</DefinedDirection><Source>ReferenceFrame</Source><SourceDirection>+Z</SourceDirection><FeatureName></FeatureName></SecondaryAxis></Value></Frame></Frames>  MarkerShape=Sphere  MarkerSize=10  GraphicType=FromGeometry  InertiaType=CalculateFromGeometry  Mass=1  MassUnits=kg  MomentsOfInertia=[1 1 1]  MomentsOfInertiaUnits=kg*m^2  GraphicOpacity=1.0  ProductsOfInertia=[0 0 0]  ProductsOfInertiaUnits=kg*m^2  GraphicShininess=75  GraphicSpecularColor=[0.5 0.5 0.5 1.0]  GraphicVisPropType=SimpleVisualProperties
  hip : sm_lib/Joints/Revolute Joint  JointMode=Normal  SenseConstraintForce=off  SenseConstraintForceX=off  SenseConstraintForceY=off  SenseConstraintForceZ=off  SenseConstraintTorque=off  SenseConstraintTorqueX=off  SenseConstraintTorqueY=off  SenseConstraintTorqueZ=off  SenseTotalForce=off  SenseTotalForceX=off  SenseTotalForceY=off  SenseTotalForceZ=off  SenseTotalTorque=off  SenseTotalTorqueX=off  SenseTotalTorqueY=off  SenseTotalTorqueZ=off  CompositeWrenchDir=FollowerOnBase  CompositeWrenchFrame=BaseFrame  EquilibriumPosition=0  EquilibriumPositionUnits=deg  SpringStiffness=0  SpringStiffnessUnits=N*m/deg  DampingCoefficient=0  DampingCoefficientUnits=N*m/(deg/s)  TorqueActuationMode=InputTorque  MotionActuationMode=ComputedMotion  SensePosition=on  SenseVelocity=on  SenseAcceleration=off  SenseTorqueForce=off  SenseLowerLimitTorqueForce=off  SenseUpperLimitTorqueForce=off  LowerLimitSpecify=off  LowerLimitBound=-90  LowerLimitBoundUnits=deg  LowerLimitStiffness=1e4  LowerLimitStiffnessUnits=N*m/deg  LowerLimitDamping=10  LowerLimitDampingUnits=N*m/(deg/s)  LowerLimitTransitionRegionWidth=0.1  LowerLimitTransitionRegionWidthUnits=deg  UpperLimitSpecify=off  UpperLimitBound=90  UpperLimitBoundUnits=deg  UpperLimitStiffness=1e4  UpperLimitStiffnessUnits=N*m/deg  UpperLimitDamping=10  UpperLimitDampingUnits=N*m/(deg/s)  UpperLimitTransitionRegionWidth=0.1  UpperLimitTransitionRegionWidthUnits=deg  PositionTargetSpecify=off  PositionTargetPriority=High  PositionTargetValue=0  PositionTargetValueUnits=deg  VelocityTargetSpecify=off  VelocityTargetPriority=High  VelocityTargetValue=0  VelocityTargetValueUnits=deg/s
  hip_dq : nesl_utility/PS-Simulink Converter  PhysicalDomain=network_engine_domain  SubClassName=ps_output  LeftPortType=input  RightPortType=output  PseudoPeriodic=off  Frequencies=[]  VectorFormat=inherit  Unit=inherit  AffineConversion=off
  hip_q : nesl_utility/PS-Simulink Converter  PhysicalDomain=network_engine_domain  SubClassName=ps_output  LeftPortType=input  RightPortType=output  PseudoPeriodic=off  Frequencies=[]  VectorFormat=inherit  Unit=inherit  AffineConversion=off
  link1 : sm_lib/Body Elements/Brick Solid  GraphicAmbientColor=[0.15 0.15 0.15 1.0]  BasedOnType=Mass  BrickDimensions=[0.2 0.05 0.05]  BrickDimensionsUnits=m  CenterOfMass=[0 0 0]  CenterOfMassUnits=m  GraphicDiffuseColor=[0.5 0.5 0.5]  Density=1000  DensityUnits=kg/m^3  DoExposeReferenceFrame=on  GraphicEmissiveColor=[0.0 0.0 0.0 1.0]  ExportEntireGeometry=off  SerializedFrames=<Frames><Frame><Id>Frame1</Id><Value><Name>thigh</Name><Origin><Source>GeometricFeature</Source><FeatureName>+x surface</FeatureName></Origin><PrimaryAxis><DefinedDirection>+Z</DefinedDirection><Source>ReferenceFrame</Source><SourceDirection>+X</SourceDirection><FeatureName></FeatureName></PrimaryAxis><SecondaryAxis><DefinedDirection>+X</DefinedDirection><Source>ReferenceFrame</Source><SourceDirection>-Z</SourceDirection><FeatureName></FeatureName></SecondaryAxis></Value></Frame></Frames>  MarkerShape=Sphere  MarkerSize=10  GraphicType=FromGeometry  InertiaType=CalculateFromGeometry  Mass=0.2  MassUnits=kg  MomentsOfInertia=[1 1 1]  MomentsOfInertiaUnits=kg*m^2  GraphicOpacity=1.0  ProductsOfInertia=[0 0 0]  ProductsOfInertiaUnits=kg*m^2  GraphicShininess=75  GraphicSpecularColor=[0.5 0.5 0.5 1.0]  GraphicVisPropType=SimpleVisualProperties
  shank : sm_lib/Body Elements/Brick Solid  GraphicAmbientColor=[0.15 0.15 0.15 1.0]  BasedOnType=Mass  BrickDimensions=[0.07 0.8 0.07]  BrickDimensionsUnits=m  CenterOfMass=[0 0 0]  CenterOfMassUnits=m  GraphicDiffuseColor=[0.5 0.5 0.5]  Density=1000  DensityUnits=kg/m^3  DoExposeReferenceFrame=on  GraphicEmissiveColor=[0.0 0.0 0.0 1.0]  ExportEntireGeometry=off  SerializedFrames=<Frames><Frame><Id>Frame1</Id><Value><Name>F1</Name><Origin><Source>GeometricFeature</Source><FeatureName>-y surface</FeatureName></Origin><PrimaryAxis><DefinedDirection>+Z</DefinedDirection><Source>ReferenceFrame</Source><SourceDirection>+Z</SourceDirection><FeatureName></FeatureName></PrimaryAxis><SecondaryAxis><DefinedDirection>+X</DefinedDirection><Source>ReferenceFrame</Source><SourceDirection>+X</SourceDirection><FeatureName></FeatureName></SecondaryAxis></Value></Frame></Frames>  MarkerShape=Sphere  MarkerSize=10  GraphicType=FromGeometry  InertiaType=CalculateFromGeometry  Mass=0.5  MassUnits=kg  MomentsOfInertia=[1 1 1]  MomentsOfInertiaUnits=kg*m^2  GraphicOpacity=1.0  ProductsOfInertia=[0 0 0]  ProductsOfInertiaUnits=kg*m^2  GraphicShininess=75  GraphicSpecularColor=[0.5 0.5 0.5 1.0]  GraphicVisPropType=SimpleVisualProperties
  shank_dq : nesl_utility/PS-Simulink Converter  PhysicalDomain=network_engine_domain  SubClassName=ps_output  LeftPortType=input  RightPortType=output  PseudoPeriodic=off  Frequencies=[]  VectorFormat=inherit  Unit=inherit  AffineConversion=off
  shank_q : nesl_utility/PS-Simulink Converter  PhysicalDomain=network_engine_domain  SubClassName=ps_output  LeftPortType=input  RightPortType=output  PseudoPeriodic=off  Frequencies=[]  VectorFormat=inherit  Unit=inherit  AffineConversion=off
  thigh : sm_lib/Body Elements/Brick Solid  GraphicAmbientColor=[0.15 0.15 0.15 1.0]  BasedOnType=Mass  BrickDimensions=[0.07 0.8 0.07]  BrickDimensionsUnits=m  CenterOfMass=[0 0 0]  CenterOfMassUnits=m  GraphicDiffuseColor=[0.5 0.5 0.5]  Density=1000  DensityUnits=kg/m^3  DoExposeReferenceFrame=on  GraphicEmissiveColor=[0.0 0.0 0.0 1.0]  ExportEntireGeometry=off  SerializedFrames=<Frames><Frame><Id>Frame1</Id><Value><Name>F1</Name><Origin><Source>GeometricFeature</Source><FeatureName>-y surface</FeatureName></Origin><PrimaryAxis><DefinedDirection>+Z</DefinedDirection><Source>ReferenceFrame</Source><SourceDirection>+Z</SourceDirection><FeatureName></FeatureName></PrimaryAxis><SecondaryAxis><DefinedDirection>+Y</DefinedDirection><Source>ReferenceFrame</Source><SourceDirection>+Y</SourceDirection><FeatureName></FeatureName></SecondaryAxis></Value></Frame></Frames>  MarkerShape=Sphere  MarkerSize=10  GraphicType=FromGeometry  InertiaType=CalculateFromGeometry  Mass=0.5  MassUnits=kg  MomentsOfInertia=[1 1 1]  MomentsOfInertiaUnits=kg*m^2  GraphicOpacity=1.0  ProductsOfInertia=[0 0 0]  ProductsOfInertiaUnits=kg*m^2  GraphicShininess=75  GraphicSpecularColor=[0.5 0.5 0.5 1.0]  GraphicVisPropType=SimpleVisualProperties
  thigh_dq : nesl_utility/PS-Simulink Converter  PhysicalDomain=network_engine_domain  SubClassName=ps_output  LeftPortType=input  RightPortType=output  PseudoPeriodic=off  Frequencies=[]  VectorFormat=inherit  Unit=inherit  AffineConversion=off
  thigh_q : nesl_utility/PS-Simulink Converter  PhysicalDomain=network_engine_domain  SubClassName=ps_output  LeftPortType=input  RightPortType=output  PseudoPeriodic=off  Frequencies=[]  VectorFormat=inherit  Unit=inherit  AffineConversion=off
  tip : sm_lib/Body Elements/Spherical Solid  GraphicAmbientColor=[0.15 0.15 0.15 1.0]  BasedOnType=Mass  CenterOfMass=[0 0 0]  CenterOfMassUnits=m  GraphicDiffuseColor=[0.0 1.0 0.6]  Density=1000  DensityUnits=kg/m^3  DoExposeReferenceFrame=on  GraphicEmissiveColor=[0.0 0.0 0.0 1.0]  ExportEntireGeometry=on  SerializedExposedGeometries=<exposedGeometries><exposedGeom><rawGeomId>entire</rawGeomId><exposedGeomId>G</exposedGeomId></exposedGeom></exposedGeometries>  SerializedFrames=<Frames/>  MarkerShape=Sphere  MarkerSize=10  GraphicType=FromGeometry  InertiaType=CalculateFromGeometry  Mass=0.01  MassUnits=kg  MomentsOfInertia=[1 1 1]  MomentsOfInertiaUnits=kg*m^2  GraphicOpacity=1.0  ProductsOfInertia=[0 0 0]  ProductsOfInertiaUnits=kg*m^2  GraphicShininess=75  GraphicSpecularColor=[0.5 0.5 0.5 1.0]  SphereRadius=0.08  SphereRadiusUnits=m  GraphicVisPropType=SimpleVisualProperties
  tiptouch : PMIOPort  Side=Left
  hipcon : PMIOPort  Port=2  Side=Left
  states : Outport
  wires:
  Bus Creator/1 -> states/1
  Bus Selector/2 -> Simulink-PS Converter1/1  "<tq2>"
  thigh_q/1 -> Bus Creator/2
  thigh_dq/1 -> Bus Creator/5
  hip_q/1 -> Bus Creator/1
  Bus Selector/1 -> Simulink-PS Converter/1  "<tq1>"
  hip_dq/1 -> Bus Creator/4
  Bus Selector/3 -> Simulink-PS Converter2/1  "<tq3>"
  shank_dq/1 -> Bus Creator/6
  shank_q/1 -> Bus Creator/3
  trqs/1 -> Bus Selector/1
  connections:
  tip/LConn1 -- tiptouch/RConn1
  Revolute Joint1/RConn3 -- shank_dq/LConn1
  Revolute Joint1/RConn2 -- shank_q/LConn1
  Simulink-PS Converter2/RConn1 -- Revolute Joint1/LConn2
  Revolute Joint/RConn2 -- thigh_q/LConn1
  Simulink-PS Converter/RConn1 -- hip/LConn2
  hip/RConn3 -- hip_dq/LConn1
  base/LConn1 -- hip/LConn1
  hip/RConn1 -- Rigid Transform/LConn1
  Simulink-PS Converter1/RConn1 -- Revolute Joint/LConn2
  hip/RConn2 -- hip_q/LConn1
  link1/RConn1 -- Rigid Transform/RConn1
  Revolute Joint1/LConn1 -- thigh/LConn1
  Rigid Transform3/LConn1 -- Revolute Joint1/RConn1
  thigh/RConn1 -- Rigid Transform2/RConn1
  Rigid Transform3/RConn1 -- shank/RConn1
  Revolute Joint/RConn3 -- thigh_dq/LConn1
  Revolute Joint/RConn1 -- Rigid Transform2/LConn1
  Rigid Transform4/LConn1 -- hipcon/RConn1
  shank/LConn1 -- tip/RConn1
  Rigid Transform4/RConn1 -- base/RConn1
  link1/LConn1 -- Revolute Joint/LConn1
